simulink model "practica2arx"  (Simulink 5.0)
settings: Solver=ode45  StartTime=0.0  StopTime=140  RelTol=1e-3
undefined symbols (not defined in the file): ts
libraries: simulink x6, dspstat3 x4
settings Model: LastModifiedBy=pc1  BlockReductionOpt=off  BooleanDataType=off

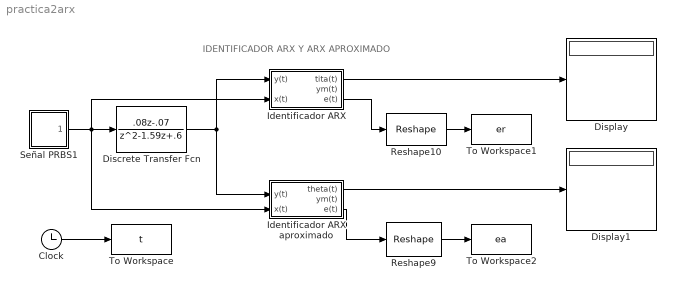
== system practica2arx ==
  note: IDENTIFICADOR ARX Y ARX APROXIMADO
  Clock : Clock
      settings: Decimation=10
  Discrete Transfer Fcn : DiscreteTransferFcn  Numerator=[.08 -.07]  Denominator=[1 -1.59 .6]  SampleTime=ts
  Display : Display
  Display1 : Display
  Identificador ARX : Subsystem  mask{l=.8, ts=ts, nk=0, nb=2, na=2}
      mask prompts: l "valor landa"; ts "valor ts"; nk "valor nk"; nb "valor nb"; na "Valor na"
  Identificador ARX aproximado : Subsystem  mask{s=.0009, ts=ts, nk=0, nb=2, na=2}
      mask prompts: s "Valor de sencivilidad u(t)"; ts "valor ts"; nk "valor nk"; nb "valor nb"; na "Valor na"
  Reshape10 : simulink/Math Operations/Reshape  OutputDimensionality=1-D array  OutputDimensions=[1,1]
  Reshape9 : simulink/Math Operations/Reshape  OutputDimensionality=1-D array  OutputDimensions=[1,1]
  Señal PRBS1 : Subsystem
  To Workspace : ToWorkspace  VariableName=t  SampleTime=-1  SaveFormat=Array
  To Workspace1 : ToWorkspace  VariableName=er  SampleTime=-1  SaveFormat=Array
  To Workspace2 : ToWorkspace  VariableName=ea  SampleTime=-1  SaveFormat=Array
  wires:
  Señal PRBS1/1(u ( t )) -> Discrete Transfer Fcn/1, Identificador ARX aproximado/2(x(t)), Identificador ARX/2(x(t))
  Identificador ARX aproximado/1(theta(t)) -> Display1/1
  Discrete Transfer Fcn/1 -> Identificador ARX/1(y(t)), Identificador ARX aproximado/1(y(t))
  Identificador ARX/3(e(t)) -> Reshape10/1
  Clock/1 -> To Workspace/1
  Identificador ARX aproximado/3(e(t)) -> Reshape9/1
  Reshape9/1 -> To Workspace2/1
  Reshape10/1 -> To Workspace1/1
  Identificador ARX/1(tita(t)) -> Display/1

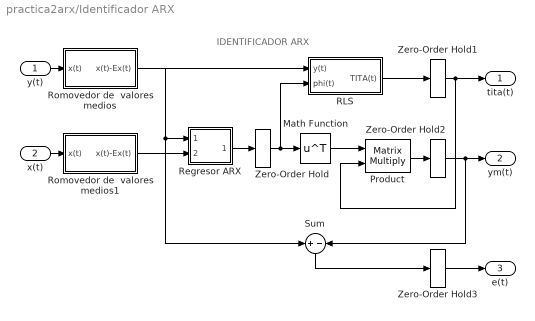
== system practica2arx/Identificador ARX ==
  note: IDENTIFICADOR ARX
  y(t) : Inport
  x(t) : Inport  Port=2
  Math Function : Math  Operator=transpose
  Product : Product  Multiplication=Matrix(*)  SaturateOnIntegerOverflow=on  InputSameDT=on
  RLS : Subsystem
  Regresor ARX : Subsystem
  Romovedor de  valores medios : Subsystem
  Romovedor de  valores medios1 : Subsystem
  Sum : Sum  Orientation=down  Inputs=+-  SaturateOnIntegerOverflow=on  InputSameDT=on
  Zero-Order Hold{,1..3} (4 alike) : ZeroOrderHold  SampleTime=ts
  tita(t) : Outport
  ym(t) : Outport  Port=2
  e(t) : Outport  Port=3
  wires:
  Math Function/1 -> Product/1
  Zero-Order Hold3/1 -> e(t)/1
  Product/1 -> Zero-Order Hold2/1
  Zero-Order Hold1/1 -> tita(t)/1, Product/2
  Zero-Order Hold/1 -> RLS/2(phi(t)), Math Function/1
  RLS/1(TITA(t)) -> Zero-Order Hold1/1
  x(t)/1 -> Romovedor de  valores medios1/1(x(t))
  y(t)/1 -> Romovedor de  valores medios/1(x(t))
  Romovedor de  valores medios/1(x(t)-Ex(t)) -> RLS/1(y(t)), Regresor ARX/1(y(t)), Sum/1
  Romovedor de  valores medios1/1(x(t)-Ex(t)) -> Regresor ARX/2(u(t))
  Regresor ARX/1(phi) -> Zero-Order Hold/1
  Zero-Order Hold2/1 -> ym(t)/1, Sum/2
  Sum/1 -> Zero-Order Hold3/1

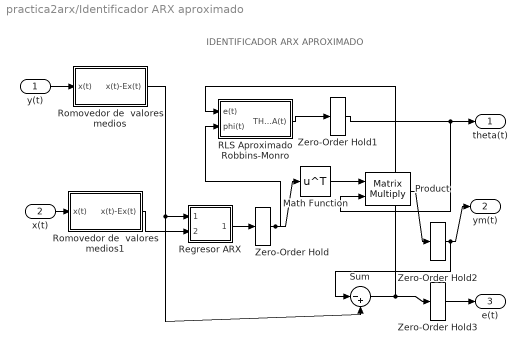
== system practica2arx/Identificador ARX aproximado ==
  note: IDENTIFICADOR ARX APROXIMADO
  y(t) : Inport
  x(t) : Inport  Port=2
  Math Function : Math  Operator=transpose
  Product : Product  Multiplication=Matrix(*)  SaturateOnIntegerOverflow=on  InputSameDT=on
  RLS Aproximado Robbins-Monro : Subsystem
  Regresor ARX : Subsystem
  Romovedor de  valores medios : Subsystem
  Romovedor de  valores medios1 : Subsystem
  Sum : Sum  Inputs=|-+  SaturateOnIntegerOverflow=on  InputSameDT=on
  Zero-Order Hold{,1..3} (4 alike) : ZeroOrderHold  SampleTime=ts
  theta(t) : Outport
  ym(t) : Outport  Port=2
  e(t) : Outport  Port=3
  wires:
  Regresor ARX/1(phi) -> Zero-Order Hold/1
  Romovedor de  valores medios1/1(x(t)-Ex(t)) -> Regresor ARX/2(u(t))
  Romovedor de  valores medios/1(x(t)-Ex(t)) -> Regresor ARX/1(y(t)), Sum/2
  y(t)/1 -> Romovedor de  valores medios/1(x(t))
  x(t)/1 -> Romovedor de  valores medios1/1(x(t))
  RLS Aproximado Robbins-Monro/1(THETA(t)) -> Zero-Order Hold1/1
  Zero-Order Hold/1 -> RLS Aproximado Robbins-Monro/2(phi(t)), Math Function/1
  Zero-Order Hold1/1 -> Product/2, theta(t)/1
  Product/1 -> Zero-Order Hold2/1
  Zero-Order Hold2/1 -> ym(t)/1, Sum/1
  Sum/1 -> RLS Aproximado Robbins-Monro/1(e(t)), Zero-Order Hold3/1
  Zero-Order Hold3/1 -> e(t)/1
  Math Function/1 -> Product/1

== system practica2arx/Señal PRBS1 ==
  Random Number : RandomNumber  SampleTime=0
  Sign : Signum
  Zero-Order Hold : ZeroOrderHold  SampleTime=ts
  u ( t ) : Outport
  wires:
  Zero-Order Hold/1 -> u ( t )/1
  Sign/1 -> Zero-Order Hold/1
  Random Number/1 -> Sign/1

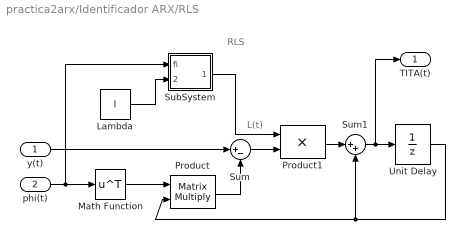
== system practica2arx/Identificador ARX/RLS ==
  note: RLS
  note: L(t)
  y(t) : Inport
  phi(t) : Inport  Port=2
  Lambda : Constant  Value=l
  Math Function : Math  Operator=transpose
  Product : Product  Multiplication=Matrix(*)  SaturateOnIntegerOverflow=on  InputSameDT=on
  Product1 : Product  SaturateOnIntegerOverflow=on  InputSameDT=on
  SubSystem : Subsystem
  Sum : Sum  Inputs=|+-  SaturateOnIntegerOverflow=on  InputSameDT=on
  Sum1 : Sum  Inputs=|++  SaturateOnIntegerOverflow=on  InputSameDT=on
  Unit Delay : UnitDelay  X0=zeros(1,na+nb)'  SampleTime=ts
  TITA(t) : Outport
  wires:
  phi(t)/1 -> SubSystem/1(fi), Math Function/1
  Math Function/1 -> Product/1
  Unit Delay/1 -> Product/2, Sum1/2
  Product/1 -> Sum/2
  y(t)/1 -> Sum/1
  Sum/1 -> Product1/2
  SubSystem/1(L(t)) -> Product1/1
  Lambda/1 -> SubSystem/2(landa)
  Sum1/1 -> Unit Delay/1, TITA(t)/1
  Product1/1 -> Sum1/1

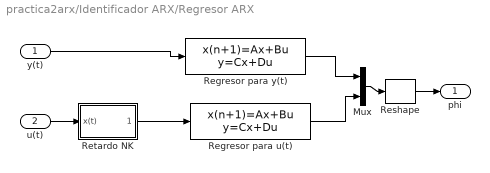
== system practica2arx/Identificador ARX/Regresor ARX ==
  y(t) : Inport
  u(t) : Inport  Port=2
  Mux : Mux  Inputs=2
  Regresor para u(t) : DiscreteStateSpace  A=[zeros(1,nb);eye(nb-1,nb)]  B=[1,zeros(1,nb-1)]'  C=eye(nb)  D=[zeros(nb,1)]  SampleTime=ts
  Regresor para y(t) : DiscreteStateSpace  A=[zeros(1,na);eye(na-1,na)]  B=[-1,zeros(1,na-1)]'  C=eye(na)  D=[zeros(na,1)]  SampleTime=ts
  Reshape : simulink/Math Operations/Reshape  OutputDimensionality=Column vector  OutputDimensions=[1,1]
  Retardo NK : Subsystem  mask{nk=nk}
      mask prompts: nk "Valor nk"
  phi : Outport
  wires:
  Reshape/1 -> phi/1
  Retardo NK/1(x(t-nk)) -> Regresor para u(t)/1
  u(t)/1 -> Retardo NK/1(x(t))
  Mux/1 -> Reshape/1
  y(t)/1 -> Regresor para y(t)/1
  Regresor para u(t)/1 -> Mux/2
  Regresor para y(t)/1 -> Mux/1

== system practica2arx/Identificador ARX/Romovedor de  valores medios ==
  x(t) : Inport
  Mean : dspstat3/Mean  run=on  reset_popup=None
  Sum : Sum  Inputs=|-+  SaturateOnIntegerOverflow=on  InputSameDT=on
  Zero-Order Hold : ZeroOrderHold  SampleTime=ts
  x(t)-Ex(t) : Outport
  wires:
  x(t)/1 -> Zero-Order Hold/1
  Zero-Order Hold/1 -> Mean/1, Sum/2
  Mean/1 -> Sum/1
  Sum/1 -> x(t)-Ex(t)/1

== system practica2arx/Identificador ARX/Romovedor de  valores medios1 ==
  x(t) : Inport
  Mean : dspstat3/Mean  run=on  reset_popup=None
  Sum : Sum  Inputs=|-+  SaturateOnIntegerOverflow=on  InputSameDT=on
  Zero-Order Hold : ZeroOrderHold  SampleTime=ts
  x(t)-Ex(t) : Outport
  wires:
  x(t)/1 -> Zero-Order Hold/1
  Zero-Order Hold/1 -> Mean/1, Sum/2
  Mean/1 -> Sum/1
  Sum/1 -> x(t)-Ex(t)/1

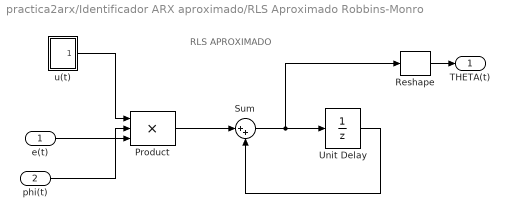
== system practica2arx/Identificador ARX aproximado/RLS Aproximado Robbins-Monro ==
  note: RLS APROXIMADO
  e(t) : Inport
  phi(t) : Inport  Port=2
  Product : Product  Inputs=3  SaturateOnIntegerOverflow=on  InputSameDT=on
  Reshape : simulink/Math Operations/Reshape  OutputDimensionality=Column vector  OutputDimensions=[1,1]
  Sum : Sum  Inputs=|++  SaturateOnIntegerOverflow=on  InputSameDT=on
  Unit Delay : UnitDelay  X0=zeros(1,na+nb)'  SampleTime=ts
  u(t) : Subsystem
  THETA(t) : Outport
  wires:
  e(t)/1 -> Product/3
  phi(t)/1 -> Product/2
  u(t)/1(u(t)) -> Product/1
  Product/1 -> Sum/1
  Unit Delay/1 -> Sum/2
  Sum/1 -> Reshape/1, Unit Delay/1
  Reshape/1 -> THETA(t)/1

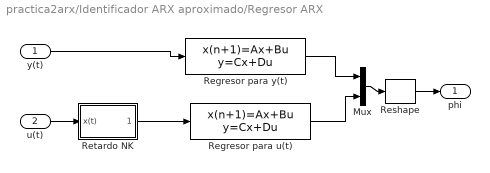
== system practica2arx/Identificador ARX aproximado/Regresor ARX ==
  y(t) : Inport
  u(t) : Inport  Port=2
  Mux : Mux  Inputs=2
  Regresor para u(t) : DiscreteStateSpace  A=[zeros(1,nb);eye(nb-1,nb)]  B=[1,zeros(1,nb-1)]'  C=eye(nb)  D=[zeros(nb,1)]  SampleTime=ts
  Regresor para y(t) : DiscreteStateSpace  A=[zeros(1,na);eye(na-1,na)]  B=[-1,zeros(1,na-1)]'  C=eye(na)  D=[zeros(na,1)]  SampleTime=ts
  Reshape : simulink/Math Operations/Reshape  OutputDimensionality=Column vector  OutputDimensions=[1,1]
  Retardo NK : Subsystem  mask{nk=nk}
      mask prompts: nk "Valor nk"
  phi : Outport
  wires:
  Regresor para y(t)/1 -> Mux/1
  Regresor para u(t)/1 -> Mux/2
  y(t)/1 -> Regresor para y(t)/1
  Mux/1 -> Reshape/1
  u(t)/1 -> Retardo NK/1(x(t))
  Retardo NK/1(x(t-nk)) -> Regresor para u(t)/1
  Reshape/1 -> phi/1

== system practica2arx/Identificador ARX aproximado/Romovedor de  valores medios ==
  x(t) : Inport
  Mean : dspstat3/Mean  run=on  reset_popup=None
  Sum : Sum  Inputs=|-+  SaturateOnIntegerOverflow=on  InputSameDT=on
  Zero-Order Hold : ZeroOrderHold  SampleTime=ts
  x(t)-Ex(t) : Outport
  wires:
  Sum/1 -> x(t)-Ex(t)/1
  Mean/1 -> Sum/1
  Zero-Order Hold/1 -> Sum/2, Mean/1
  x(t)/1 -> Zero-Order Hold/1

== system practica2arx/Identificador ARX aproximado/Romovedor de  valores medios1 ==
  x(t) : Inport
  Mean : dspstat3/Mean  run=on  reset_popup=None
  Sum : Sum  Inputs=|-+  SaturateOnIntegerOverflow=on  InputSameDT=on
  Zero-Order Hold : ZeroOrderHold  SampleTime=ts
  x(t)-Ex(t) : Outport
  wires:
  Sum/1 -> x(t)-Ex(t)/1
  Mean/1 -> Sum/1
  Zero-Order Hold/1 -> Sum/2, Mean/1
  x(t)/1 -> Zero-Order Hold/1

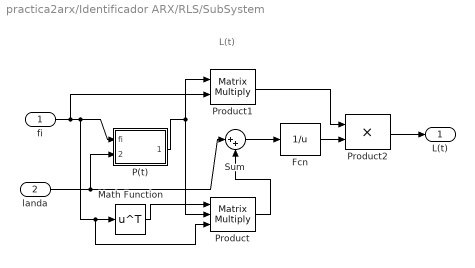
== system practica2arx/Identificador ARX/RLS/SubSystem ==
  note: L(t)
  fi : Inport
  landa : Inport  Port=2
  Fcn : Fcn  Expr=1/u
  Math Function : Math  Operator=transpose
  P(t) : Subsystem
  Product : Product  Inputs=3  Multiplication=Matrix(*)  SaturateOnIntegerOverflow=on  InputSameDT=on
  Product1 : Product  Multiplication=Matrix(*)  SaturateOnIntegerOverflow=on  InputSameDT=on
  Product2 : Product  SaturateOnIntegerOverflow=on  InputSameDT=on
  Sum : Sum  Inputs=|++  SaturateOnIntegerOverflow=on  InputSameDT=on
  L(t) : Outport
  wires:
  Product2/1 -> L(t)/1
  P(t)/1(P(t-1)) -> Product/2, Product1/1
  fi/1 -> P(t)/1(fi), Math Function/1, Product/3, Product1/2
  landa/1 -> P(t)/2(landa), Sum/1
  Math Function/1 -> Product/1
  Product/1 -> Sum/2
  Sum/1 -> Fcn/1
  Fcn/1 -> Product2/2
  Product1/1 -> Product2/1

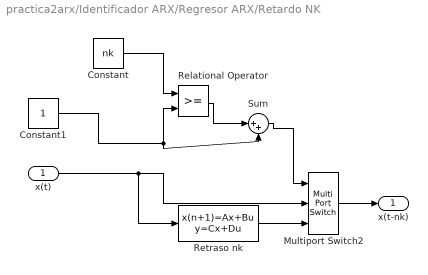
== system practica2arx/Identificador ARX/Regresor ARX/Retardo NK ==
  x(t) : Inport
  Constant : Constant  Value=nk
  Constant1 : Constant
  Multiport Switch2 : MultiPortSwitch  Inputs=2  SaturateOnIntegerOverflow=on  InputSameDT=on
  Relational Operator : RelationalOperator  InputSameDT=on
  Retraso nk : DiscreteStateSpace  A=[zeros(1,max(nk,1));eye(max(nk,1)-1,max(nk,1))]  B=[1,zeros(1,max(nk,1)-1)]'  C=[zeros(1,max(nk,1)-1),1]  D=[0]  SampleTime=ts
  Sum : Sum  Inputs=|++  SaturateOnIntegerOverflow=on  InputSameDT=on
  x(t-nk) : Outport
  wires:
  x(t)/1 -> Retraso nk/1, Multiport Switch2/2
  Multiport Switch2/1 -> x(t-nk)/1
  Retraso nk/1 -> Multiport Switch2/3
  Sum/1 -> Multiport Switch2/1
  Relational Operator/1 -> Sum/1
  Constant/1 -> Relational Operator/1
  Constant1/1 -> Sum/2, Relational Operator/2

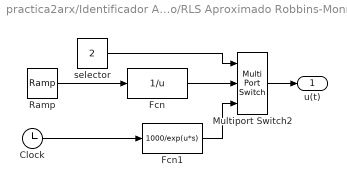
== system practica2arx/Identificador ARX aproximado/RLS Aproximado Robbins-Monro/u(t) ==
  Clock : Clock
      settings: Decimation=10
  Fcn : Fcn  Expr=1/u
  Fcn1 : Fcn  Expr=1000/exp(u*s)
  Multiport Switch2 : MultiPortSwitch  Inputs=2  SaturateOnIntegerOverflow=on  InputSameDT=on
  Ramp : simulink/Sources/Ramp  slope=s  start=0  X0=1
  selector : Constant  Value=2
  u(t) : Outport
  wires:
  Ramp/1 -> Fcn/1
  Clock/1 -> Fcn1/1
  Fcn/1 -> Multiport Switch2/2
  Fcn1/1 -> Multiport Switch2/3
  Multiport Switch2/1 -> u(t)/1
  selector/1 -> Multiport Switch2/1

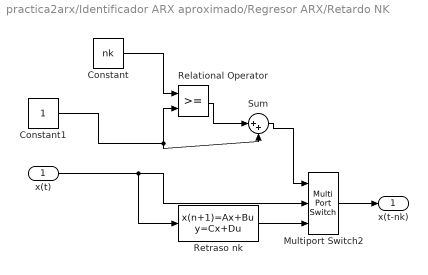
== system practica2arx/Identificador ARX aproximado/Regresor ARX/Retardo NK ==
  x(t) : Inport
  Constant : Constant  Value=nk
  Constant1 : Constant
  Multiport Switch2 : MultiPortSwitch  Inputs=2  SaturateOnIntegerOverflow=on  InputSameDT=on
  Relational Operator : RelationalOperator  InputSameDT=on
  Retraso nk : DiscreteStateSpace  A=[zeros(1,max(nk,1));eye(max(nk,1)-1,max(nk,1))]  B=[1,zeros(1,max(nk,1)-1)]'  C=[zeros(1,max(nk,1)-1),1]  D=[0]  SampleTime=ts
  Sum : Sum  Inputs=|++  SaturateOnIntegerOverflow=on  InputSameDT=on
  x(t-nk) : Outport
  wires:
  Constant1/1 -> Relational Operator/2, Sum/2
  Constant/1 -> Relational Operator/1
  Relational Operator/1 -> Sum/1
  Sum/1 -> Multiport Switch2/1
  Retraso nk/1 -> Multiport Switch2/3
  Multiport Switch2/1 -> x(t-nk)/1
  x(t)/1 -> Multiport Switch2/2, Retraso nk/1

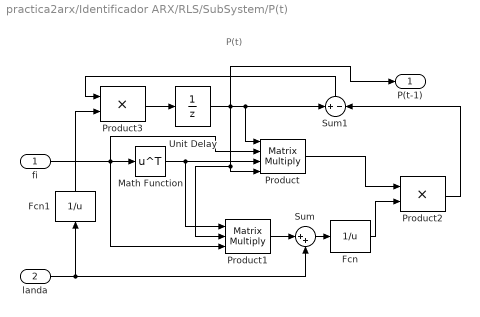
== system practica2arx/Identificador ARX/RLS/SubSystem/P(t) ==
  note: P(t)
  fi : Inport
  landa : Inport  Port=2
  Fcn : Fcn  Expr=1/u
  Fcn1 : Fcn  Orientation=up  Expr=1/u
  Math Function : Math  Operator=transpose
  Product : Product  Inputs=4  Multiplication=Matrix(*)  SaturateOnIntegerOverflow=on  InputSameDT=on
  Product1 : Product  Inputs=3  Multiplication=Matrix(*)  SaturateOnIntegerOverflow=on  InputSameDT=on
  Product2 : Product  SaturateOnIntegerOverflow=on  InputSameDT=on
  Product3 : Product  SaturateOnIntegerOverflow=on  InputSameDT=on
  Sum : Sum  Inputs=|++  SaturateOnIntegerOverflow=on  InputSameDT=on
  Sum1 : Sum  Orientation=up  Inputs=+-  SaturateOnIntegerOverflow=on  InputSameDT=on
  Unit Delay : UnitDelay  X0=100000*eye(na+nb)  SampleTime=ts
  P(t-1) : Outport
  wires:
  Fcn1/1 -> Product3/2
  fi/1 -> Math Function/1, Product/2, Product1/3
  Unit Delay/1 -> P(t-1)/1, Product/4, Product1/2, Product/1, Sum1/1
  Math Function/1 -> Product/3, Product1/1
  Product1/1 -> Sum/1
  landa/1 -> Fcn1/1, Sum/2
  Sum/1 -> Fcn/1
  Fcn/1 -> Product2/2
  Product/1 -> Product2/1
  Sum1/1 -> Product3/1
  Product3/1 -> Unit Delay/1
  Product2/1 -> Sum1/2
